simulink model "Neuro_schema"  (Simulink 7.7)
settings: Solver=ode45  StartTime=0.0  StopTime=2  RelTol=1e-3
undefined symbols (not defined in the file or in its folder): quad
libraries: simulink x4, neural x1
settings Model: Creator=Alexey  LastModifiedBy=Alexey

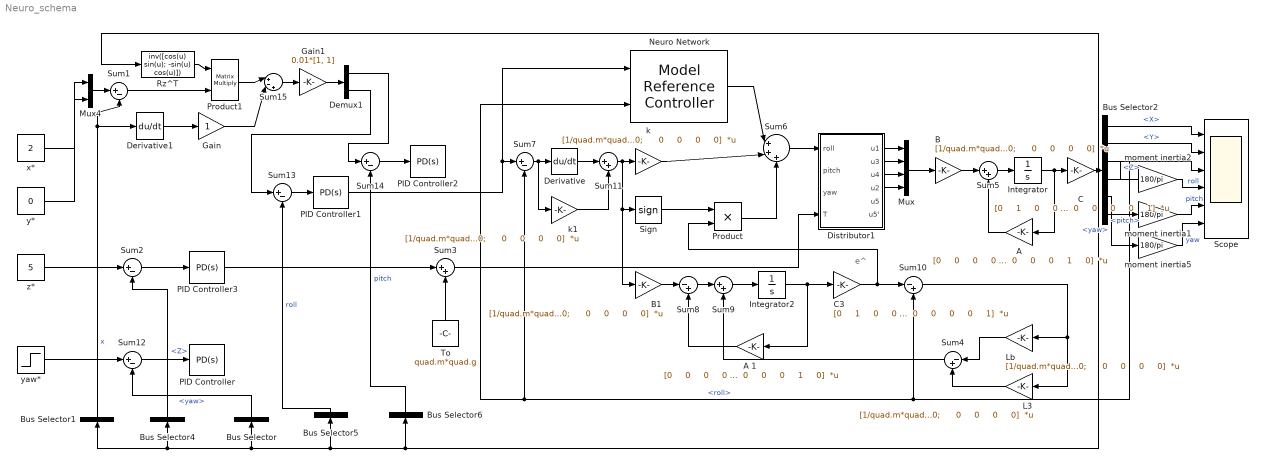
== system Neuro_schema ==
  note: e^
  "A " : Gain  Gain=|  Multiplication=Matrix(K*u)
      | [0     0     0     0     0     0     0     0;
      |      1     0     0     0     0     0     0     0;
      |      0     0     0     0     0     0     0     0;
      |      0     0     1     0     0     0     0     0;
      |      0     0     0     0     0     0     0     0;
      |      0     0     0     0     1     0     0     0;
      |      0     0     0     0     0     0     0     0;
      |      0     0     0     0     0     0     1     0]
  A 1 : Gain  Gain=|  Multiplication=Matrix(K*u)
      | [0     0     0     0     0     0     0     0;
      |      1     0     0     0     0     0     0     0;
      |      0     0     0     0     0     0     0     0;
      |      0     0     1     0     0     0     0     0;
      |      0     0     0     0     0     0     0     0;
      |      0     0     0     0     1     0     0     0;
      |      0     0     0     0     0     0     0     0;
      |      0     0     0     0     0     0     1     0]
  B : Gain  Gain=|  Multiplication=Matrix(K*u)
      | [1/quad.m*quad.b     0     0     0;
      |      0     0     0     0;
      |      0     0     1/quad.Ixx*quad.b*quad.l     0;
      |      0     0     0     0;
      |      0     0     0     1/quad.Iyy*quad.b*quad.l;
      |      0     0     0     0;
      |      0     1/quad.Izz*quad.k     0     0;
      |      0     0     0     0]
  B1 : Gain  Gain=|  Multiplication=Matrix(K*u)
      | [1/quad.m*quad.b     0     0     0;
      |      0     0     0     0;
      |      0     0     1/quad.Ixx*quad.b*quad.l     0;
      |      0     0     0     0;
      |      0     0     0     1/quad.Iyy*quad.b*quad.l;
      |      0     0     0     0;
      |      0     1/quad.Izz*quad.k*quad.r     0     0;
      |      0     0     0     0]
  Bus Selector : BusSelector  OutputSignals=yaw
  Bus Selector1 : BusSelector  OutputSignals=X,Y  OutputAsBus=on
  Bus Selector2 : BusSelector  OutputSignals=X,Y,Z,roll,pitch,yaw
  Bus Selector4 : BusSelector  OutputSignals=Z
  Bus Selector5 : BusSelector  OutputSignals=roll  OutputAsBus=on
  Bus Selector6 : BusSelector  OutputSignals=pitch  OutputAsBus=on
  C : Gain  Gain=|  Multiplication=Matrix(K*u)
      | [0     1     0     0     0     0     0     0;
      |      0     0     0     1     0     0     0     0;
      |      0     0     0     0     0     1     0     0;
      |      0     0     0     0     0     0     0     1]
  C3 : Gain  Gain=|  Multiplication=Matrix(K*u)
      | [0     1     0     0     0     0     0     0;
      |      0     0     0     1     0     0     0     0;
      |      0     0     0     0     0     1     0     0;
      |      0     0     0     0     0     0     0     1]
  Demux1 : Demux  Outputs=2
  Derivative : Derivative
  Derivative1 : Derivative
  Distributor1 : Subsystem
  Gain : Gain
  Gain1 : Gain  Gain=0.01*[1, 1]
  Integrator : Integrator
  Integrator2 : Integrator
  L3 : Gain  Gain=|  Multiplication=Matrix(K*u)
      | [1/quad.m*quad.b     0     0     0;
      |      0     0     0     0;
      |      0     0     1/quad.Ixx*quad.b*quad.l     0;
      |      0     0     0     0;
      |      0     0     0     1/quad.Iyy*quad.b*quad.l;
      |      0     0     0     0;
      |      0     1/quad.Izz*quad.k*quad.r     0     0;
      |      0     0     0     0]
  Lb : Gain  Gain=|  Multiplication=Matrix(K*u)
      | [1/quad.m*quad.b     0     0     0;
      |      0     0     0     0;
      |      0     0     1/quad.Ixx*quad.b*quad.l     0;
      |      0     0     0     0;
      |      0     0     0     1/quad.Iyy*quad.b*quad.l;
      |      0     0     0     0;
      |      0     1/quad.Izz*quad.k*quad.r     0     0;
      |      0     0     0     0]
  Mux : Mux
  Mux4 : Mux  Inputs=2
  Neuro Network : neural/Control Systems/Model Reference Controller  SystemSampleTime=-1  trainfun=trainlm
  PID Controller : simulink/Continuous/PID Controller  SystemSampleTime=-1  Controller=PD  TimeDomain=Continuous-time  SampleTime=1  IntegratorMethod=Forward Euler  FilterMethod=Forward Euler  Form=Parallel  P=1  I=1  D=1  N=100  InitialConditionSource=internal  InitialConditionForIntegrator=0  InitialConditionForFilter=0  ExternalReset=none  LimitOutput=off  UpperSaturationLimit=inf  LowerSaturationLimit=-inf  LinearizeAsGain=off  AntiWindupMode=none  Kb=1  TrackingMode=off  Kt=1  PParamMin=[]  PParamMax=[]  IParamMin=[]  IParamMax=[]  DParamMin=[]  DParamMax=[]  NParamMin=[]  NParamMax=[]  KbParamMin=[]  KbParamMax=[]  KtParamMin=[]  KtParamMax=[]  POutMin=[]  POutMax=[]  IOutMin=[]  IOutMax=[]  DOutMin=[]  DOutMax=[]  NOutMin=[]  NOutMax=[]  KbOutMin=[]  KbOutMax=[]  KtOutMin=[]  KtOutMax=[]  IntegratorOutMin=[]  IntegratorOutMax=[]  FilterOutMin=[]  FilterOutMax=[]  SumOutMin=[]  SumOutMax=[]  SumI1OutMin=[]  SumI1OutMax=[]  SumI2OutMin=[]  SumI2OutMax=[]  SumI3OutMin=[]  SumI3OutMax=[]  SumDOutMin=[]  SumDOutMax=[]  SaturationOutMin=[]  SaturationOutMax=[]  IntegratorContinuousStateAttributes=''  IntegratorStateMustResolveToSignalObject=off  IntegratorRTWStateStorageClass=Auto  FilterContinuousStateAttributes=''  FilterStateMustResolveToSignalObject=off  FilterRTWStateStorageClass=Auto
  PID Controller1 : simulink/Continuous/PID Controller  SystemSampleTime=-1  Controller=PD  TimeDomain=Continuous-time  SampleTime=1  IntegratorMethod=Forward Euler  FilterMethod=Forward Euler  Form=Parallel  P=1  I=0  D=1  N=100  InitialConditionSource=internal  InitialConditionForIntegrator=0  InitialConditionForFilter=0  ExternalReset=none  LimitOutput=off  UpperSaturationLimit=inf  LowerSaturationLimit=-inf  LinearizeAsGain=off  AntiWindupMode=none  Kb=1  TrackingMode=off  Kt=1  PParamMin=[]  PParamMax=[]  IParamMin=[]  IParamMax=[]  DParamMin=[]  DParamMax=[]  NParamMin=[]  NParamMax=[]  KbParamMin=[]  KbParamMax=[]  KtParamMin=[]  KtParamMax=[]  POutMin=[]  POutMax=[]  IOutMin=[]  IOutMax=[]  DOutMin=[]  DOutMax=[]  NOutMin=[]  NOutMax=[]  KbOutMin=[]  KbOutMax=[]  KtOutMin=[]  KtOutMax=[]  IntegratorOutMin=[]  IntegratorOutMax=[]  FilterOutMin=[]  FilterOutMax=[]  SumOutMin=[]  SumOutMax=[]  SumI1OutMin=[]  SumI1OutMax=[]  SumI2OutMin=[]  SumI2OutMax=[]  SumI3OutMin=[]  SumI3OutMax=[]  SumDOutMin=[]  SumDOutMax=[]  SaturationOutMin=[]  SaturationOutMax=[]  IntegratorContinuousStateAttributes=''  IntegratorStateMustResolveToSignalObject=off  IntegratorRTWStateStorageClass=Auto  FilterContinuousStateAttributes=''  FilterStateMustResolveToSignalObject=off  FilterRTWStateStorageClass=Auto
  PID Controller2 : simulink/Continuous/PID Controller  SystemSampleTime=-1  Controller=PD  TimeDomain=Continuous-time  SampleTime=1  IntegratorMethod=Forward Euler  FilterMethod=Forward Euler  Form=Parallel  P=1  I=0  D=1  N=100  InitialConditionSource=internal  InitialConditionForIntegrator=0  InitialConditionForFilter=0  ExternalReset=none  LimitOutput=off  UpperSaturationLimit=inf  LowerSaturationLimit=-inf  LinearizeAsGain=off  AntiWindupMode=none  Kb=1  TrackingMode=off  Kt=1  PParamMin=[]  PParamMax=[]  IParamMin=[]  IParamMax=[]  DParamMin=[]  DParamMax=[]  NParamMin=[]  NParamMax=[]  KbParamMin=[]  KbParamMax=[]  KtParamMin=[]  KtParamMax=[]  POutMin=[]  POutMax=[]  IOutMin=[]  IOutMax=[]  DOutMin=[]  DOutMax=[]  NOutMin=[]  NOutMax=[]  KbOutMin=[]  KbOutMax=[]  KtOutMin=[]  KtOutMax=[]  IntegratorOutMin=[]  IntegratorOutMax=[]  FilterOutMin=[]  FilterOutMax=[]  SumOutMin=[]  SumOutMax=[]  SumI1OutMin=[]  SumI1OutMax=[]  SumI2OutMin=[]  SumI2OutMax=[]  SumI3OutMin=[]  SumI3OutMax=[]  SumDOutMin=[]  SumDOutMax=[]  SaturationOutMin=[]  SaturationOutMax=[]  IntegratorContinuousStateAttributes=''  IntegratorStateMustResolveToSignalObject=off  IntegratorRTWStateStorageClass=Auto  FilterContinuousStateAttributes=''  FilterStateMustResolveToSignalObject=off  FilterRTWStateStorageClass=Auto
  PID Controller3 : simulink/Continuous/PID Controller  SystemSampleTime=-1  Controller=PD  TimeDomain=Continuous-time  SampleTime=1  IntegratorMethod=Forward Euler  FilterMethod=Forward Euler  Form=Parallel  P=1  I=1  D=1.5  N=100  InitialConditionSource=internal  InitialConditionForIntegrator=0  InitialConditionForFilter=0  ExternalReset=none  LimitOutput=off  UpperSaturationLimit=inf  LowerSaturationLimit=-inf  LinearizeAsGain=off  AntiWindupMode=none  Kb=1  TrackingMode=off  Kt=1  PParamMin=[]  PParamMax=[]  IParamMin=[]  IParamMax=[]  DParamMin=[]  DParamMax=[]  NParamMin=[]  NParamMax=[]  KbParamMin=[]  KbParamMax=[]  KtParamMin=[]  KtParamMax=[]  POutMin=[]  POutMax=[]  IOutMin=[]  IOutMax=[]  DOutMin=[]  DOutMax=[]  NOutMin=[]  NOutMax=[]  KbOutMin=[]  KbOutMax=[]  KtOutMin=[]  KtOutMax=[]  IntegratorOutMin=[]  IntegratorOutMax=[]  FilterOutMin=[]  FilterOutMax=[]  SumOutMin=[]  SumOutMax=[]  SumI1OutMin=[]  SumI1OutMax=[]  SumI2OutMin=[]  SumI2OutMax=[]  SumI3OutMin=[]  SumI3OutMax=[]  SumDOutMin=[]  SumDOutMax=[]  SaturationOutMin=[]  SaturationOutMax=[]  IntegratorContinuousStateAttributes=''  IntegratorStateMustResolveToSignalObject=off  IntegratorRTWStateStorageClass=Auto  FilterContinuousStateAttributes=''  FilterStateMustResolveToSignalObject=off  FilterRTWStateStorageClass=Auto
  Product : Product  RndMeth=Zero
  Product1 : Product  Multiplication=Matrix(*)  RndMeth=Zero
  Rz^T : MATLABFcn  MATLABFcn=inv([cos(u) sin(u); -sin(u) cos(u)])  OutputDimensions=[2 2]  Output1D=off
  Scope : Scope  NumInputPorts=6
      settings: TimeRange=2  YMin=-500~0~-1~-225~-30~-1000  YMax=100~800~1~-75~20~7000
  Sign : Signum
  Sum{1..2,7,12..14} (6 alike) : Sum  Inputs=|+-
  Sum10 : Sum  Inputs=|-+
  Sum{3,5,9,11} (4 alike) : Sum  Inputs=|++
  Sum15 : Sum  Inputs=|+-+
  Sum4 : Sum  Inputs=|-+
  Sum6 : Sum  Inputs=|+++
  Sum8 : Sum  Inputs=|-+
  To : Constant  Value=quad.m*quad.g
  k : Gain  Gain=|  Multiplication=Matrix(K*u)
      | [1/quad.m*quad.b     0     0     0;
      |      0     0     0     0;
      |      0     0     1/quad.Ixx*quad.b*quad.l     0;
      |      0     0     0     0;
      |      0     0     0     1/quad.Iyy*quad.b*quad.l;
      |      0     0     0     0;
      |      0     1/quad.Izz*quad.k     0     0;
      |      0     0     0     0]
  k1 : Gain  Gain=|  Multiplication=Matrix(K*u)
      | [1/quad.m*quad.b     0     0     0;
      |      0     0     0     0;
      |      0     0     1/quad.Ixx*quad.b*quad.l     0;
      |      0     0     0     0;
      |      0     0     0     1/quad.Iyy*quad.b*quad.l;
      |      0     0     0     0;
      |      0     1/quad.Izz*quad.k     0     0;
      |      0     0     0     0]
  moment inertia1 : Gain  Gain=180/pi
  moment inertia2 : Gain  Gain=180/pi
  moment inertia5 : Gain  Gain=180/pi
  x* : Constant  Value=2
  y* : Constant  Value=0
  yaw* : Step  Time=10  Before=0*pi/180  After=0*pi/180  SampleTime=0
  z* : Constant  Value=5
  wires:
  B/1 -> Sum5/1
  Sum5/1 -> Integrator/1
  Integrator/1 -> C/1, "A "/1
  "A "/1 -> Sum5/2
  Mux/1 -> B/1
  Distributor1/1("u1 ") -> Mux/1
  Distributor1/4("u2 ") -> Mux/4
  Distributor1/2("u3 ") -> Mux/2
  Distributor1/3("u4 ") -> Mux/3
  Neuro Network/1 -> Sum6/1
  k/1 -> Sum6/2
  Sign/1 -> Product/1
  Product/1 -> Sum6/3
  Sum6/1 -> Distributor1/1(roll)
  B1/1 -> Sum8/1
  A 1/1 -> Sum8/2
  Sum8/1 -> Sum9/1
  Sum9/1 -> Integrator2/1
  Integrator2/1 -> C3/1, A 1/1
  C3/1 -> Sum10/1, Product/2
  C/1 -> Rz^T/1, Bus Selector6/1, Bus Selector4/1, Bus Selector1/1, Bus Selector/1, Bus Selector5/1, Bus Selector2/1
  Sum7/1 -> Derivative/1, k1/1
  Derivative/1 -> Sum11/1
  Sum11/1 -> k/1, Sign/1, B1/1
  k1/1 -> Sum11/2
  Lb/1 -> Sum4/1
  L3/1 -> Sum4/2
  Sum10/1 -> Lb/1, L3/1
  Sum4/1 -> Sum9/2
  x*/1 -> Mux4/1
  y*/1 -> Mux4/2
  Bus Selector/1 -> Sum12/2  "<yaw>"
  Bus Selector1/1 -> Sum1/2, Derivative1/1  "x"
  Bus Selector5/1 -> Sum13/2  "roll"
  Bus Selector4/1 -> Sum2/2  "<Z>"
  Bus Selector6/1 -> Sum14/2  "pitch"
  To/1 -> Sum3/2
  z*/1 -> Sum2/1
  Sum2/1 -> PID Controller3/1
  yaw*/1 -> Sum12/1
  Sum12/1 -> PID Controller/1
  Sum13/1 -> PID Controller1/1
  Demux1/1 -> Sum14/1
  Sum14/1 -> PID Controller2/1
  Sum3/1 -> Distributor1/4(T)
  PID Controller1/1 -> Sum7/1, Neuro Network/1
  PID Controller3/1 -> Sum3/1
  Rz^T/1 -> Product1/1
  Mux4/1 -> Sum1/1
  Sum1/1 -> Product1/2
  Sum15/1 -> Gain1/1
  Product1/1 -> Sum15/1
  Derivative1/1 -> Gain/1
  Gain/1 -> Sum15/2
  Gain1/1 -> Demux1/1
  Demux1/2 -> Sum13/1
  Bus Selector2/1 -> Scope/1  "<X>"
  Bus Selector2/2 -> Scope/2  "<Y>"
  Bus Selector2/3 -> Scope/3  "<Z>"
  Bus Selector2/4 -> moment inertia2/1, Sum7/2, Neuro Network/2, Sum10/2  "<roll>"
  Bus Selector2/5 -> moment inertia1/1  "<pitch>"
  Bus Selector2/6 -> moment inertia5/1  "<yaw>"
  moment inertia5/1 -> Scope/6  "yaw"
  moment inertia1/1 -> Scope/5  "pitch"
  moment inertia2/1 -> Scope/4  "roll"

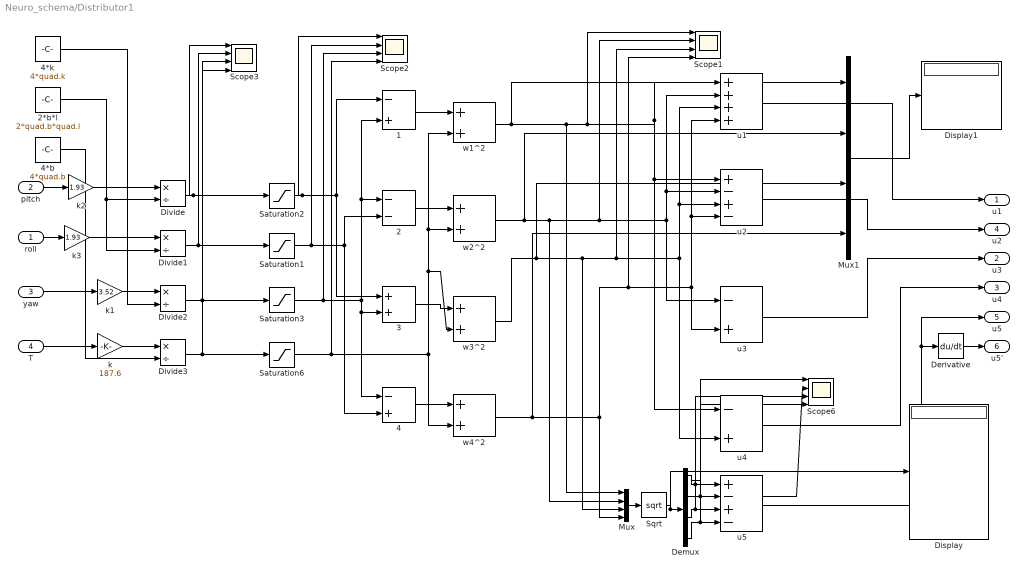
== system Neuro_schema/Distributor1 ==
  roll : Inport
  pitch : Inport  Port=2
  yaw : Inport  Port=3
  T : Inport  Port=4
  1 : Sum  Inputs=-+
  2 : Sum  Inputs=--
  2*b*l : Constant  Value=2*quad.b*quad.l
  3 : Sum
  4 : Sum  Inputs=-+
  4*b : Constant  Value=4*quad.b
  4*k : Constant  Value=4*quad.k
  Demux : Demux
  Derivative : Derivative
  Display : Display
  Display1 : Display
  Divide{,1..3} (4 alike) : Product  Inputs=*/
  Mux : Mux
  Mux1 : Mux
  Saturation1 : Saturate  UpperLimit=287850  LowerLimit=-287850
  Saturation2 : Saturate  UpperLimit=287850  LowerLimit=-287850
  Saturation3 : Saturate  UpperLimit=9000000000  LowerLimit=-9000000000  LinearizeAsGain=off
  Saturation6 : Saturate  UpperLimit=1574000000  LowerLimit=15740000
  Scope{1..3,6} (4 alike) : Scope  NumInputPorts=4
      Scope1 settings: TimeRange=1  YMin=-5~-5~-5~-5  YMax=5~5~5~5  SaveName=ScopeData2
      Scope2 settings: TimeRange=1  YMin=-5~-5~-5~-5  YMax=5~5~5~5  SaveName=ScopeData4
      Scope3 settings: TimeRange=1  YMin=-5~-5~-5~-5  YMax=5~5~5~5  SaveName=ScopeData5
      Scope6 settings: TimeRange=1  YMin=-5~-5~-5~-5  YMax=5~5~5~5  SaveName=ScopeData6
  Sqrt : Sqrt  SaturateOnIntegerOverflow=on
  k : Gain  Gain=187.6
  k1 : Gain  Gain=3.52
  k2 : Gain  Gain=1.93
  k3 : Gain  Gain=1.93
  u1 : Sum  Inputs=++++
  u2 : Sum  Inputs=+-+-
  u3 : Sum  Inputs=-+
  u4 : Sum  Inputs=-+
  u5 : Sum  Inputs=+-+-
  w1^2 : Sum
  w2^2 : Sum
  w3^2 : Sum
  w4^2 : Sum
  "u1 " : Outport
  "u3 " : Outport  Port=2
  "u4 " : Outport  Port=3
  "u2 " : Outport  Port=4
  "u5 " : Outport  Port=5
  u5' : Outport  Port=6
  wires:
  4*k/1 -> Divide2/2
  Divide1/1 -> Scope3/2, Saturation1/1
  Divide2/1 -> Scope3/3, Saturation3/1
  Divide/1 -> Scope3/1, Saturation2/1
  4*b/1 -> Divide3/2
  yaw/1 -> k1/1
  2*b*l/1 -> Divide/2, Divide1/2
  roll/1 -> k3/1
  pitch/1 -> k2/1
  w1^2/1 -> Mux/1, u1/1, u2/1, u4/1, Scope1/1, Mux1/1
  w2^2/1 -> Mux/2, u1/2, u2/2, u3/1, Scope1/2, Mux1/2
  w3^2/1 -> Mux/3, u1/3, u2/3, u4/2, Scope1/3, Mux1/3
  w4^2/1 -> Mux/4, u1/4, u2/4, u3/2, Scope1/4, Mux1/4
  Divide3/1 -> Scope3/4, Saturation6/1
  T/1 -> k/1
  u1/1 -> "u1 "/1
  u2/1 -> "u2 "/1
  u3/1 -> "u3 "/1
  u4/1 -> "u4 "/1
  Mux/1 -> Sqrt/1
  Sqrt/1 -> Demux/1, Display/1
  Demux/1 -> u5/1, Scope6/1
  Demux/3 -> u5/3, Scope6/3
  Demux/2 -> u5/2, Scope6/2
  Demux/4 -> u5/4, Scope6/4
  u5/1 -> Derivative/1, "u5 "/1
  Derivative/1 -> u5'/1
  1/1 -> w1^2/1
  2/1 -> w2^2/1
  3/1 -> w3^2/1
  4/1 -> w4^2/1
  Saturation6/1 -> w1^2/2, w2^2/2, w3^2/2, w4^2/2, Scope2/4
  Mux1/1 -> Display1/1
  Saturation2/1 -> 1/1, 3/1, Scope2/1
  Saturation1/1 -> 2/2, 4/2, Scope2/2
  Saturation3/1 -> 3/2, 4/1, 1/2, 2/1, Scope2/3
  k2/1 -> Divide/1
  k3/1 -> Divide1/1
  k1/1 -> Divide2/1
  k/1 -> Divide3/1
